simulink model "Battery_Module_To_FullPack_Grouped"  (R2024b)
settings: Solver=ode23t  StartTime=0.0  StopTime=900  MaxStep=0.05  RelTol=1e-3  AbsTol=1e-3
InitFcn:
  | % Parameters
  | vec_coolant_T=module_LUTthermalData{1};
  | vec_coolant_F=module_LUTthermalData{2};
  | mat_cellQ=module_LUTthermalData{3};
  | FlwR=coolantMassFlowRate/max(vec_coolant_F);
  | FlwT=coolantTemp-ambientTemp;
undefined symbols (not defined in the file): airGapBetweenModuleLarge, airGapBetweenModuleSmall, battery_cellH, battery_cellT, battery_cellW, battery_Np, battery_Ns, endPlateThickness
libraries: fl_lib x56, nesl_utility x14, batteryModule_lib x6
(part 1 of 2)
Description:
  | Battery Pack Thermal Management
  | 
  | Copyright 2020-2024 The MathWorks, Inc.
settings Model: Creator=vikrants  LastModifiedBy=smiller
settings SolverCC: AutoScaleAbsTol=off  AlgebraicLoopSolver=TrustRegion
settings DataIOCC: ReturnWorkspaceOutputs=off  SignalLoggingName=logsout_Battery_Module_To_FullPack_Grouped
settings DebuggingCC: UnconnectedInputMsg=warning  UnconnectedOutputMsg=warning  UnconnectedLineMsg=warning  SymbolicDimsDataTypeCodeGenerationDiagnostic=none
settings ModelReferenceCC: EnableRefExpFcnMdlSchedulingChecks=on
settings SFSimCC: CustomCodeUndefinedFunction=UseInterfaceOnly
settings RTWCC: GPUComputeCapability=3.5  DLArmComputeVersion=19.05
settings SimscapeCC: SimscapeLogType=all  SimscapeLogSimulationStatistics=on  SimscapeLogName=simlog_Battery_Module_To_FullPack_Grouped  SimscapeLogDataHistory=250000

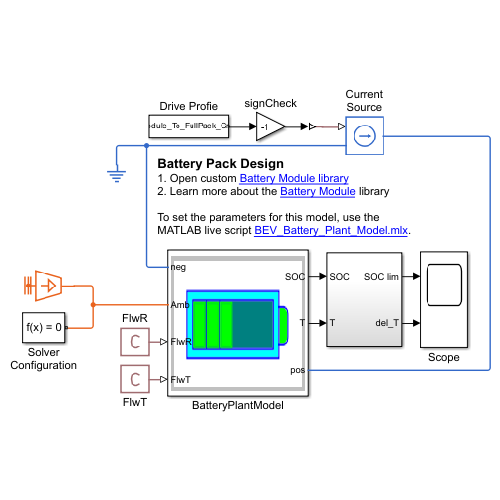
[thumbnail: Simulink's stored preview of the top-level diagram]
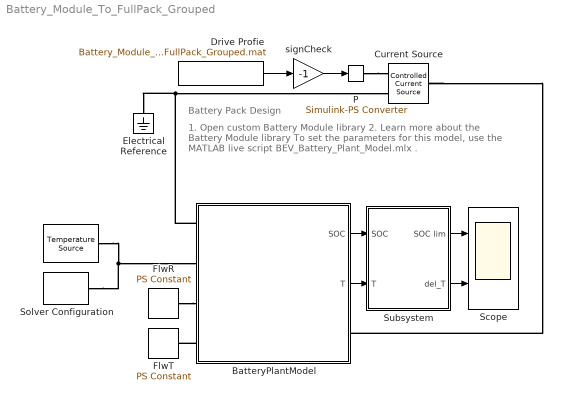
== system Battery_Module_To_FullPack_Grouped ==
  note: 1. Open custom Battery Module library
      | 2. Learn more about the Battery Module library
      |
      | To set the parameters for this model, use the
      | MATLAB live script BEV_Battery_Plant_Model.mlx .
  note: Battery Pack Design
  " " : fl_lib/Thermal/Thermal Sources/Temperature Source  temperature=ambientTemp K
  BatteryPlantModel : Subsystem
      mask Display: image('EV_Thermal_Management_BatteryIcon.png'); % Use "Edit Image" on toolstrip to change.
  Current Source : fl_lib/Electrical/Electrical Sources/Controlled Current Source
  Drive Profie : FromFile  FileName=Battery_Module_To_FullPack_Grouped.mat  SampleTime=0
  Electrical Reference : fl_lib/Electrical/Electrical Elements/Electrical Reference
  FlwR : fl_lib/Physical Signals/Sources/PS Constant  constant=FlwR
  FlwT : fl_lib/Physical Signals/Sources/PS Constant  constant=FlwT K
  P : nesl_utility/Simulink-PS Converter  PhysicalDomain=network_engine_domain  SubClassName=ps_input  LeftPortType=input  RightPortType=output  PseudoPeriodic=off  Frequencies=[]  NoiseDistribution=none  NoiseParameters=[]  Unit=A  AffineConversion=off  FilteringAndDerivatives=provide  SimscapeFilterOrder=1  InputFilterTimeConstant=0.001  UdotUserProvided=0
  Scope : Scope  NumInputPorts=2
  Solver Configuration : nesl_utility/Solver Configuration  PhysicalDomain=network_engine_domain  SubClassName=solver  LeftPortType=input  RightPortType=generic  Tones=[]  Harmonics=[]  SimulateNoise=off  Profile=off  UseLocalSampling=off  EnableSwitchedLinearOptims=on  FrequencyDomain=off  UseCCode=off  RelTol=0.001  AbsTol=1e-06  MinStep=1e-09  ToWorkspace=off  RevertToSquareIcSolve=off  NumHomotopyIterations=100  PhasorMode=off  PhasorModeNumHarmonics=1  ConsistencySolver=NEWTON_FTOL  IndexReductionMethod=DerivativeReplacement  DoDC=off  ResidualTolerance=1e-09  ConsistencyTolSource=GLOBAL  ConsistencyAbsTol=0.001  ConsistencyRelTol=0.001  ConsistencyTolFactor=0.001  UseLocalSolver=off  LocalSolverChoice=NE_BACKWARD_EULER_ADVANCER  ResolveIndetEquations=on  FunctionEvalNumThread=1  LocalSolverSampleTime=0.001  DoFixedCost=off  MaxNonlinIter=3  MaxModeIter=2  ComputeImpulses=off  ImpulseIterations=2  LinearAlgebra=auto  LinearAlgebraNumThread=0  EquationFormulation=NE_TIME_EF  DelaysMemoryBudget=1024  AutomaticFiltering=on  FilteringTimeConstant=0.001  PartitionStorageMethod=AS_NEEDED  PartitionMemoryBudget=1024  PartitionMethod=ROBUST  MultibodyUseLocalSolver=off  MultibodyLocalSolverChoice=ODE1  MultibodyLocalSolverSampleTime=0.001
  Subsystem : Subsystem
  signCheck : Gain  Gain=-1
  wires:
  Drive Profie/1 -> signCheck/1
  Subsystem/1(SOC lim) -> Scope/1
  Subsystem/2(del_T) -> Scope/2
  BatteryPlantModel/1(SOC) -> Subsystem/1(SOC)
  BatteryPlantModel/2(T) -> Subsystem/2(T)
  signCheck/1 -> P/1
  connections:
  P/RConn1 -- Current Source/RConn1
  BatteryPlantModel/LConn1 -- Electrical Reference/LConn1 -- Current Source/RConn2
  Current Source/LConn1 -- BatteryPlantModel/RConn1
  FlwR/RConn1 -- BatteryPlantModel/LConn3
  BatteryPlantModel/LConn4 -- FlwT/RConn1
  " "/LConn1 -- BatteryPlantModel/LConn2 -- Solver Configuration/RConn1

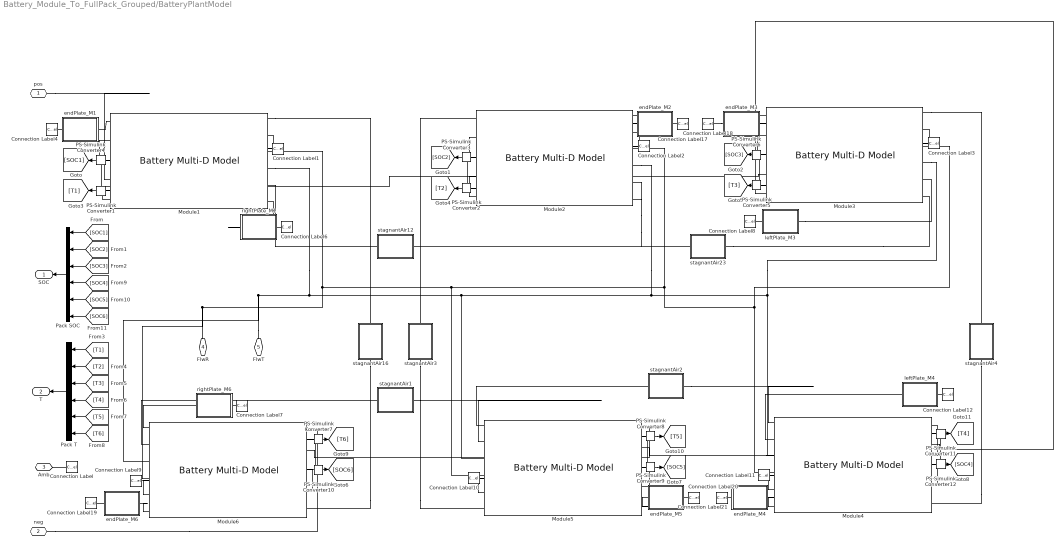
== system Battery_Module_To_FullPack_Grouped/BatteryPlantModel ==
  Connection Label{,1..4,6..12,17..21} (17 alike) : ConnectionLabel  Label=amb
  Module1 : batteryModule_lib/Battery Multi-D Model  modelComplexity=batteryModule.batteryAbstractionLevel.grouped  LUTpointsTemp=battery_vecT K  cellAH=battery_Ahr A*hr  LUTpointsSOC=battery_vecSOC  V0_mat=battery_V0 V  prm_dir=ee.enum.battery.prm_dir.noCurrentDirectionality  R0_mat=battery_R0 Ohm  R0_dis_mat=[.03, .015, .002; .04, .017, .008; .039, .012, .006; .027, .013, .021] Ohm  R0_ch_mat=[.03, .015, .002; .04, .017, .008; .039, .012, .006; .027, .013, .021] Ohm  prm_leak=ee.enum.battery.prm_leak.disabled  Rleak_vec=[8000, 7000, 6000] Ohm  extrapolation_option=simscape.enum.extrapolation.linear  prm_dyn=ee.enum.battery.prm_dyn.rc2  R1_mat=battery_R1 Ohm  tau1_mat=battery_Tau1 s  R2_mat=battery_R2 Ohm  tau2_mat=battery_Tau2 s  R3_mat=[.014, .382, .407; .028, .006, .007; .014, .007, .006; .333, .956, .912] Ohm  tau3_mat=[1, 44, 5644; 11, 24, 506; 2, 14, 330; 3310, 13419, 30216] s  R4_mat=[.014, .382, .407; .028, .006, .007; .014, .007, .006; .333, .956, .912] Ohm  tau4_mat=[1, 44, 5644; 11, 24, 506; 2, 14, 330; 3310, 13419, 30216] s  R5_mat=[.014, .382, .407; .028, .006, .007; .014, .007, .006; .333, .956, .912] Ohm  tau5_mat=[1, 44, 5644; 11, 24, 506; 2, 14, 330; 3310, 13419, 30216] s  prm_fade=ee.enum.battery.prm_fade.equations  N0=100  dV0=0  dR0=0  dAH=0  dRleak=0  dR1=0  dR2=0  dR3=0  dR4=0  dR5=0  N0vec=[100, 200, 300]  Tfadevec=[298.15, 323.15] K  dV0vec=[0, 0, 0]  dR0vec=[0, 0, 0]  dAHvec=[0, 0, 0]  dRleakvec=[0, 0, 0]  dR1vec=[0, 0, 0]  dR2vec=[0, 0, 0]  dR3vec=[0, 0, 0]  dR4vec=[0, 0, 0]  dR5vec=[0, 0, 0]  dV0mat=[0, 0; 0, 0; 0, 0]  dR0mat=[0, 0; 0, 0; 0, 0]  dAHmat=[0, 0; 0, 0; 0, 0]  dRleakmat=[0, 0; 0, 0; 0, 0]  dR1mat=[0, 0; 0, 0; 0, 0]  dR2mat=[0, 0; 0, 0; 0, 0]  dR3mat=[0, 0; 0, 0; 0, 0]  dR4mat=[0, 0; 0, 0; 0, 0]  dR5mat=[0, 0; 0, 0; 0, 0]  cellThermalMass=battery_thermalMass J/K  cellThermalCond=battery_thermalK_thru W/(m*K)  cellThermalCond_inPlane=battery_thermalK_in W/(m*K)  Ns=battery_Ns  Np=battery_Np  cellTypeSelection=batteryModule.batteryTypeSelection.pouch  cellHeight=battery_cellH m  cellWidth=battery_cellW m  cellThickness=battery_cellT m  cellDiameter=0.018 m  cellCylinLine=3  moduleExternalR=battery_extR Ohm  moduleCellBalancing=batteryModule.batteryCellBalancing.none  passiveShuntR=50 Ohm  passiveSWclosedR=0.01 Ohm  passiveSWopenCond=1e-8 1/Ohm  passiveSWthreshold=0.5  moduleCellVoltages=batteryModule.batteryCellVoltages.no  thermalManagement=batteryModule.batteryCoolingSystem.thermalPort  cellHeatTrCoeff=1 W/(m^2 * K)  thermal_moduleBottom=batteryModule.batteryThermalPortSelection.thermalLUT  htc_bottom=1 W/(m^2 * K)  moduleCooling_b=mat_cellQ W/K  LUTpointsFlowrate_b=vec_coolant_F kg/s  LUTpointsTemp_b=vec_coolant_T K  thermal_moduleTop=batteryModule.batteryThermalPortSelection.convectionBC  htc_top=battery_sidesHTC W/(m^2 * K)  moduleCooling_t=zeros(3, 6, 10) W/K  LUTpointsFlowrate_t=[.01, .02, .03, .04, .05, .06] kg/s  LUTpointsTemp_t=[273.15, 298.15, 323.15] K  thermal_moduleRight=batteryModule.batteryThermalPortSelection.thermalPortLumped  htc_right=battery_sidesHTC W/(m^2 * K)  moduleCooling_r=zeros(3, 6, 10) W/K  LUTpointsFlowrate_r=[.01, .02, .03, .04, .05, .06] kg/s  LUTpointsTemp_r=[273.15, 298.15, 323.15] K  thermal_moduleLeft=batteryModule.batteryThermalPortSelection.thermalPortLumped  htc_left=battery_sidesHTC W/(m^2 * K)  moduleCooling_l=zeros(3, 6, 10) W/K  LUTpointsFlowrate_l=[.01, .02, .03, .04, .05, .06] kg/s  LUTpointsTemp_l=[273.15, 298.15, 323.15] K  thermal_modulePos=batteryModule.batteryThermalPortSelection.thermalPortLumped  htc_pos=battery_sidesHTC W/(m^2 * K)  moduleCooling_p=zeros(3, 6, 10) W/K  LUTpointsFlowrate_p=[.01, .02, .03, .04, .05, .06] kg/s  LUTpointsTemp_p=[273.15, 298.15, 323.15] K  thermal_moduleNeg=batteryModule.batteryThermalPortSelection.thermalPortLumped  htc_neg=battery_sidesHTC W/(m^2 * K)  moduleCooling_n=zeros(3, 6, 10) W/K  LUTpointsFlowrate_n=[.01, .02, .03, .04, .05, .06] kg/s  LUTpointsTemp_n=[273.15, 298.15, 323.15] K  moduleExtHeat=battery_extHeat W  cellTemp=battery_iniT K  cellSOC=battery_iniSOC  moduleCellAHpercentVar=battery_varAhr_M1  moduleCellLeakPercentVar=ones(1, 10)  moduleCellR0PercentVar=battery_varR0_M1
      settings: InternalSimscapePortConfiguration="{\"Bottom\":[{\"id\":\"Ql\",\"label\":\"Ql\",\"type\":\"foundation.thermal.thermal\"},{\"id\":\"Qr\",\"label\":\"Qr\",\"type\":\"foundation.thermal.thermal\"}],\"Left\":[{\"id\":\"Qp\",\"label\":\"Qp\",\"type\":\"foundation.thermal.thermal\"},{\"id\":\"outputCellSOC\",\"label\":\"SOC\",\"type\":\"output\"},{\"id\":\"outputCellTemp\",\"label\":\"Temp\",\"type\":\"output\"}],\"Right\":[{\"id\":\"Qn\",\"label\":\"Qn\",\"type\":\"foundation.thermal.thermal\"},{\"id\":\"H\",\"label\":\"Amb\",\"type\":\"foundation.thermal.thermal\"},{\"id\":\"frac_b\",\"label\":\"FlwR\",\"type\":\"input\"},{\"id\":\"delT_b\",\"label\":\"FlwT\",\"type\":\"input\"}],\"Top\":[{\"id\":\"p\",\"label\":\"pos\",\"type\":\"foundation.electrical.electrical\"},{\"id\":\"n\",\"label\":\"neg\",\"type\":\"foundation.electrical.electrical\"}]}"
  Module2 : batteryModule_lib/Battery Multi-D Model  modelComplexity=batteryModule.batteryAbstractionLevel.grouped  LUTpointsTemp=battery_vecT K  cellAH=battery_Ahr A*hr  LUTpointsSOC=battery_vecSOC  V0_mat=battery_V0 V  prm_dir=ee.enum.battery.prm_dir.noCurrentDirectionality  R0_mat=battery_R0 Ohm  R0_dis_mat=[.03, .015, .002; .04, .017, .008; .039, .012, .006; .027, .013, .021] Ohm  R0_ch_mat=[.03, .015, .002; .04, .017, .008; .039, .012, .006; .027, .013, .021] Ohm  prm_leak=ee.enum.battery.prm_leak.disabled  Rleak_vec=[8000, 7000, 6000] Ohm  extrapolation_option=simscape.enum.extrapolation.linear  prm_dyn=ee.enum.battery.prm_dyn.rc2  R1_mat=battery_R1 Ohm  tau1_mat=battery_Tau1 s  R2_mat=battery_R2 Ohm  tau2_mat=battery_Tau2 s  R3_mat=[.014, .382, .407; .028, .006, .007; .014, .007, .006; .333, .956, .912] Ohm  tau3_mat=[1, 44, 5644; 11, 24, 506; 2, 14, 330; 3310, 13419, 30216] s  R4_mat=[.014, .382, .407; .028, .006, .007; .014, .007, .006; .333, .956, .912] Ohm  tau4_mat=[1, 44, 5644; 11, 24, 506; 2, 14, 330; 3310, 13419, 30216] s  R5_mat=[.014, .382, .407; .028, .006, .007; .014, .007, .006; .333, .956, .912] Ohm  tau5_mat=[1, 44, 5644; 11, 24, 506; 2, 14, 330; 3310, 13419, 30216] s  prm_fade=ee.enum.battery.prm_fade.equations  N0=100  dV0=0  dR0=0  dAH=0  dRleak=0  dR1=0  dR2=0  dR3=0  dR4=0  dR5=0  N0vec=[100, 200, 300]  Tfadevec=[298.15, 323.15] K  dV0vec=[0, 0, 0]  dR0vec=[0, 0, 0]  dAHvec=[0, 0, 0]  dRleakvec=[0, 0, 0]  dR1vec=[0, 0, 0]  dR2vec=[0, 0, 0]  dR3vec=[0, 0, 0]  dR4vec=[0, 0, 0]  dR5vec=[0, 0, 0]  dV0mat=[0, 0; 0, 0; 0, 0]  dR0mat=[0, 0; 0, 0; 0, 0]  dAHmat=[0, 0; 0, 0; 0, 0]  dRleakmat=[0, 0; 0, 0; 0, 0]  dR1mat=[0, 0; 0, 0; 0, 0]  dR2mat=[0, 0; 0, 0; 0, 0]  dR3mat=[0, 0; 0, 0; 0, 0]  dR4mat=[0, 0; 0, 0; 0, 0]  dR5mat=[0, 0; 0, 0; 0, 0]  cellThermalMass=battery_thermalMass J/K  cellThermalCond=battery_thermalK_thru W/(m*K)  cellThermalCond_inPlane=battery_thermalK_in W/(m*K)  Ns=battery_Ns  Np=battery_Np  cellTypeSelection=batteryModule.batteryTypeSelection.pouch  cellHeight=battery_cellH m  cellWidth=battery_cellW m  cellThickness=battery_cellT m  cellDiameter=0.018 m  cellCylinLine=3  moduleExternalR=battery_extR Ohm  moduleCellBalancing=batteryModule.batteryCellBalancing.none  passiveShuntR=50 Ohm  passiveSWclosedR=0.01 Ohm  passiveSWopenCond=1e-8 1/Ohm  passiveSWthreshold=0.5  moduleCellVoltages=batteryModule.batteryCellVoltages.no  thermalManagement=batteryModule.batteryCoolingSystem.thermalPort  cellHeatTrCoeff=1 W/(m^2 * K)  thermal_moduleBottom=batteryModule.batteryThermalPortSelection.thermalLUT  htc_bottom=1 W/(m^2 * K)  moduleCooling_b=mat_cellQ W/K  LUTpointsFlowrate_b=vec_coolant_F kg/s  LUTpointsTemp_b=vec_coolant_T K  thermal_moduleTop=batteryModule.batteryThermalPortSelection.convectionBC  htc_top=battery_sidesHTC W/(m^2 * K)  moduleCooling_t=zeros(3, 6, 10) W/K  LUTpointsFlowrate_t=[.01, .02, .03, .04, .05, .06] kg/s  LUTpointsTemp_t=[273.15, 298.15, 323.15] K  thermal_moduleRight=batteryModule.batteryThermalPortSelection.thermalPortLumped  htc_right=battery_sidesHTC W/(m^2 * K)  moduleCooling_r=zeros(3, 6, 10) W/K  LUTpointsFlowrate_r=[.01, .02, .03, .04, .05, .06] kg/s  LUTpointsTemp_r=[273.15, 298.15, 323.15] K  thermal_moduleLeft=batteryModule.batteryThermalPortSelection.thermalPortLumped  htc_left=battery_sidesHTC W/(m^2 * K)  moduleCooling_l=zeros(3, 6, 10) W/K  LUTpointsFlowrate_l=[.01, .02, .03, .04, .05, .06] kg/s  LUTpointsTemp_l=[273.15, 298.15, 323.15] K  thermal_modulePos=batteryModule.batteryThermalPortSelection.thermalPortLumped  htc_pos=battery_sidesHTC W/(m^2 * K)  moduleCooling_p=zeros(3, 6, 10) W/K  LUTpointsFlowrate_p=[.01, .02, .03, .04, .05, .06] kg/s  LUTpointsTemp_p=[273.15, 298.15, 323.15] K  thermal_moduleNeg=batteryModule.batteryThermalPortSelection.thermalPortLumped  htc_neg=battery_sidesHTC W/(m^2 * K)  moduleCooling_n=zeros(3, 6, 10) W/K  LUTpointsFlowrate_n=[.01, .02, .03, .04, .05, .06] kg/s  LUTpointsTemp_n=[273.15, 298.15, 323.15] K  moduleExtHeat=battery_extHeat W  cellTemp=battery_iniT K  cellSOC=battery_iniSOC  moduleCellAHpercentVar=battery_varAhr_M2  moduleCellLeakPercentVar=ones(1, 10)  moduleCellR0PercentVar=battery_varR0_M2
      settings: InternalSimscapePortConfiguration="{\"Bottom\":[{\"id\":\"Ql\",\"label\":\"Ql\",\"type\":\"foundation.thermal.thermal\"},{\"id\":\"Qr\",\"label\":\"Qr\",\"type\":\"foundation.thermal.thermal\"}],\"Left\":[{\"id\":\"Qp\",\"label\":\"Qp\",\"type\":\"foundation.thermal.thermal\"},{\"id\":\"outputCellSOC\",\"label\":\"SOC\",\"type\":\"output\"},{\"id\":\"outputCellTemp\",\"label\":\"Temp\",\"type\":\"output\"}],\"Right\":[{\"id\":\"Qn\",\"label\":\"Qn\",\"type\":\"foundation.thermal.thermal\"},{\"id\":\"H\",\"label\":\"Amb\",\"type\":\"foundation.thermal.thermal\"},{\"id\":\"frac_b\",\"label\":\"FlwR\",\"type\":\"input\"},{\"id\":\"delT_b\",\"label\":\"FlwT\",\"type\":\"input\"}],\"Top\":[{\"id\":\"p\",\"label\":\"pos\",\"type\":\"foundation.electrical.electrical\"},{\"id\":\"n\",\"label\":\"neg\",\"type\":\"foundation.electrical.electrical\"}]}"
  Module3 : batteryModule_lib/Battery Multi-D Model  modelComplexity=batteryModule.batteryAbstractionLevel.grouped  LUTpointsTemp=battery_vecT K  cellAH=battery_Ahr A*hr  LUTpointsSOC=battery_vecSOC  V0_mat=battery_V0 V  prm_dir=ee.enum.battery.prm_dir.noCurrentDirectionality  R0_mat=battery_R0 Ohm  R0_dis_mat=[.03, .015, .002; .04, .017, .008; .039, .012, .006; .027, .013, .021] Ohm  R0_ch_mat=[.03, .015, .002; .04, .017, .008; .039, .012, .006; .027, .013, .021] Ohm  prm_leak=ee.enum.battery.prm_leak.disabled  Rleak_vec=[8000, 7000, 6000] Ohm  extrapolation_option=simscape.enum.extrapolation.linear  prm_dyn=ee.enum.battery.prm_dyn.rc2  R1_mat=battery_R1 Ohm  tau1_mat=battery_Tau1 s  R2_mat=battery_R2 Ohm  tau2_mat=battery_Tau2 s  R3_mat=[.014, .382, .407; .028, .006, .007; .014, .007, .006; .333, .956, .912] Ohm  tau3_mat=[1, 44, 5644; 11, 24, 506; 2, 14, 330; 3310, 13419, 30216] s  R4_mat=[.014, .382, .407; .028, .006, .007; .014, .007, .006; .333, .956, .912] Ohm  tau4_mat=[1, 44, 5644; 11, 24, 506; 2, 14, 330; 3310, 13419, 30216] s  R5_mat=[.014, .382, .407; .028, .006, .007; .014, .007, .006; .333, .956, .912] Ohm  tau5_mat=[1, 44, 5644; 11, 24, 506; 2, 14, 330; 3310, 13419, 30216] s  prm_fade=ee.enum.battery.prm_fade.equations  N0=100  dV0=0  dR0=0  dAH=0  dRleak=0  dR1=0  dR2=0  dR3=0  dR4=0  dR5=0  N0vec=[100, 200, 300]  Tfadevec=[298.15, 323.15] K  dV0vec=[0, 0, 0]  dR0vec=[0, 0, 0]  dAHvec=[0, 0, 0]  dRleakvec=[0, 0, 0]  dR1vec=[0, 0, 0]  dR2vec=[0, 0, 0]  dR3vec=[0, 0, 0]  dR4vec=[0, 0, 0]  dR5vec=[0, 0, 0]  dV0mat=[0, 0; 0, 0; 0, 0]  dR0mat=[0, 0; 0, 0; 0, 0]  dAHmat=[0, 0; 0, 0; 0, 0]  dRleakmat=[0, 0; 0, 0; 0, 0]  dR1mat=[0, 0; 0, 0; 0, 0]  dR2mat=[0, 0; 0, 0; 0, 0]  dR3mat=[0, 0; 0, 0; 0, 0]  dR4mat=[0, 0; 0, 0; 0, 0]  dR5mat=[0, 0; 0, 0; 0, 0]  cellThermalMass=battery_thermalMass J/K  cellThermalCond=battery_thermalK_thru W/(m*K)  cellThermalCond_inPlane=battery_thermalK_in W/(m*K)  Ns=battery_Ns  Np=battery_Np  cellTypeSelection=batteryModule.batteryTypeSelection.pouch  cellHeight=battery_cellH m  cellWidth=battery_cellW m  cellThickness=battery_cellT m  cellDiameter=0.018 m  cellCylinLine=3  moduleExternalR=battery_extR Ohm  moduleCellBalancing=batteryModule.batteryCellBalancing.none  passiveShuntR=50 Ohm  passiveSWclosedR=0.01 Ohm  passiveSWopenCond=1e-8 1/Ohm  passiveSWthreshold=0.5  moduleCellVoltages=batteryModule.batteryCellVoltages.no  thermalManagement=batteryModule.batteryCoolingSystem.thermalPort  cellHeatTrCoeff=1 W/(m^2 * K)  thermal_moduleBottom=batteryModule.batteryThermalPortSelection.thermalLUT  htc_bottom=1 W/(m^2 * K)  moduleCooling_b=mat_cellQ W/K  LUTpointsFlowrate_b=vec_coolant_F kg/s  LUTpointsTemp_b=vec_coolant_T K  thermal_moduleTop=batteryModule.batteryThermalPortSelection.convectionBC  htc_top=battery_sidesHTC W/(m^2 * K)  moduleCooling_t=zeros(3, 6, 10) W/K  LUTpointsFlowrate_t=[.01, .02, .03, .04, .05, .06] kg/s  LUTpointsTemp_t=[273.15, 298.15, 323.15] K  thermal_moduleRight=batteryModule.batteryThermalPortSelection.thermalPortLumped  htc_right=battery_sidesHTC W/(m^2 * K)  moduleCooling_r=zeros(3, 6, 10) W/K  LUTpointsFlowrate_r=[.01, .02, .03, .04, .05, .06] kg/s  LUTpointsTemp_r=[273.15, 298.15, 323.15] K  thermal_moduleLeft=batteryModule.batteryThermalPortSelection.thermalPortLumped  htc_left=battery_sidesHTC W/(m^2 * K)  moduleCooling_l=zeros(3, 6, 10) W/K  LUTpointsFlowrate_l=[.01, .02, .03, .04, .05, .06] kg/s  LUTpointsTemp_l=[273.15, 298.15, 323.15] K  thermal_modulePos=batteryModule.batteryThermalPortSelection.thermalPortLumped  htc_pos=battery_sidesHTC W/(m^2 * K)  moduleCooling_p=zeros(3, 6, 10) W/K  LUTpointsFlowrate_p=[.01, .02, .03, .04, .05, .06] kg/s  LUTpointsTemp_p=[273.15, 298.15, 323.15] K  thermal_moduleNeg=batteryModule.batteryThermalPortSelection.thermalPortLumped  htc_neg=battery_sidesHTC W/(m^2 * K)  moduleCooling_n=zeros(3, 6, 10) W/K  LUTpointsFlowrate_n=[.01, .02, .03, .04, .05, .06] kg/s  LUTpointsTemp_n=[273.15, 298.15, 323.15] K  moduleExtHeat=battery_extHeat W  cellTemp=battery_iniT K  cellSOC=battery_iniSOC  moduleCellAHpercentVar=battery_varAhr_M3  moduleCellLeakPercentVar=ones(1, 10)  moduleCellR0PercentVar=battery_varR0_M3
      settings: InternalSimscapePortConfiguration="{\"Bottom\":[{\"id\":\"Ql\",\"label\":\"Ql\",\"type\":\"foundation.thermal.thermal\"},{\"id\":\"Qr\",\"label\":\"Qr\",\"type\":\"foundation.thermal.thermal\"}],\"Left\":[{\"id\":\"Qp\",\"label\":\"Qp\",\"type\":\"foundation.thermal.thermal\"},{\"id\":\"outputCellSOC\",\"label\":\"SOC\",\"type\":\"output\"},{\"id\":\"outputCellTemp\",\"label\":\"Temp\",\"type\":\"output\"}],\"Right\":[{\"id\":\"Qn\",\"label\":\"Qn\",\"type\":\"foundation.thermal.thermal\"},{\"id\":\"H\",\"label\":\"Amb\",\"type\":\"foundation.thermal.thermal\"},{\"id\":\"frac_b\",\"label\":\"FlwR\",\"type\":\"input\"},{\"id\":\"delT_b\",\"label\":\"FlwT\",\"type\":\"input\"}],\"Top\":[{\"id\":\"p\",\"label\":\"pos\",\"type\":\"foundation.electrical.electrical\"},{\"id\":\"n\",\"label\":\"neg\",\"type\":\"foundation.electrical.electrical\"}]}"
  Module4 : batteryModule_lib/Battery Multi-D Model  modelComplexity=batteryModule.batteryAbstractionLevel.grouped  LUTpointsTemp=battery_vecT K  cellAH=battery_Ahr A*hr  LUTpointsSOC=battery_vecSOC  V0_mat=battery_V0 V  prm_dir=ee.enum.battery.prm_dir.noCurrentDirectionality  R0_mat=battery_R0 Ohm  R0_dis_mat=[.03, .015, .002; .04, .017, .008; .039, .012, .006; .027, .013, .021] Ohm  R0_ch_mat=[.03, .015, .002; .04, .017, .008; .039, .012, .006; .027, .013, .021] Ohm  prm_leak=ee.enum.battery.prm_leak.disabled  Rleak_vec=[8000, 7000, 6000] Ohm  extrapolation_option=simscape.enum.extrapolation.linear  prm_dyn=ee.enum.battery.prm_dyn.rc2  R1_mat=battery_R1 Ohm  tau1_mat=battery_Tau1 s  R2_mat=battery_R2 Ohm  tau2_mat=battery_Tau2 s  R3_mat=[.014, .382, .407; .028, .006, .007; .014, .007, .006; .333, .956, .912] Ohm  tau3_mat=[1, 44, 5644; 11, 24, 506; 2, 14, 330; 3310, 13419, 30216] s  R4_mat=[.014, .382, .407; .028, .006, .007; .014, .007, .006; .333, .956, .912] Ohm  tau4_mat=[1, 44, 5644; 11, 24, 506; 2, 14, 330; 3310, 13419, 30216] s  R5_mat=[.014, .382, .407; .028, .006, .007; .014, .007, .006; .333, .956, .912] Ohm  tau5_mat=[1, 44, 5644; 11, 24, 506; 2, 14, 330; 3310, 13419, 30216] s  prm_fade=ee.enum.battery.prm_fade.equations  N0=100  dV0=0  dR0=0  dAH=0  dRleak=0  dR1=0  dR2=0  dR3=0  dR4=0  dR5=0  N0vec=[100, 200, 300]  Tfadevec=[298.15, 323.15] K  dV0vec=[0, 0, 0]  dR0vec=[0, 0, 0]  dAHvec=[0, 0, 0]  dRleakvec=[0, 0, 0]  dR1vec=[0, 0, 0]  dR2vec=[0, 0, 0]  dR3vec=[0, 0, 0]  dR4vec=[0, 0, 0]  dR5vec=[0, 0, 0]  dV0mat=[0, 0; 0, 0; 0, 0]  dR0mat=[0, 0; 0, 0; 0, 0]  dAHmat=[0, 0; 0, 0; 0, 0]  dRleakmat=[0, 0; 0, 0; 0, 0]  dR1mat=[0, 0; 0, 0; 0, 0]  dR2mat=[0, 0; 0, 0; 0, 0]  dR3mat=[0, 0; 0, 0; 0, 0]  dR4mat=[0, 0; 0, 0; 0, 0]  dR5mat=[0, 0; 0, 0; 0, 0]  cellThermalMass=battery_thermalMass J/K  cellThermalCond=battery_thermalK_thru W/(m*K)  cellThermalCond_inPlane=battery_thermalK_in W/(m*K)  Ns=battery_Ns  Np=battery_Np  cellTypeSelection=batteryModule.batteryTypeSelection.pouch  cellHeight=battery_cellH m  cellWidth=battery_cellW m  cellThickness=battery_cellT m  cellDiameter=0.018 m  cellCylinLine=3  moduleExternalR=battery_extR Ohm  moduleCellBalancing=batteryModule.batteryCellBalancing.none  passiveShuntR=50 Ohm  passiveSWclosedR=0.01 Ohm  passiveSWopenCond=1e-8 1/Ohm  passiveSWthreshold=0.5  moduleCellVoltages=batteryModule.batteryCellVoltages.no  thermalManagement=batteryModule.batteryCoolingSystem.thermalPort  cellHeatTrCoeff=1 W/(m^2 * K)  thermal_moduleBottom=batteryModule.batteryThermalPortSelection.thermalLUT  htc_bottom=1 W/(m^2 * K)  moduleCooling_b=mat_cellQ W/K  LUTpointsFlowrate_b=vec_coolant_F kg/s  LUTpointsTemp_b=vec_coolant_T K  thermal_moduleTop=batteryModule.batteryThermalPortSelection.convectionBC  htc_top=battery_sidesHTC W/(m^2 * K)  moduleCooling_t=zeros(3, 6, 10) W/K  LUTpointsFlowrate_t=[.01, .02, .03, .04, .05, .06] kg/s  LUTpointsTemp_t=[273.15, 298.15, 323.15] K  thermal_moduleRight=batteryModule.batteryThermalPortSelection.thermalPortLumped  htc_right=battery_sidesHTC W/(m^2 * K)  moduleCooling_r=zeros(3, 6, 10) W/K  LUTpointsFlowrate_r=[.01, .02, .03, .04, .05, .06] kg/s  LUTpointsTemp_r=[273.15, 298.15, 323.15] K  thermal_moduleLeft=batteryModule.batteryThermalPortSelection.thermalPortLumped  htc_left=battery_sidesHTC W/(m^2 * K)  moduleCooling_l=zeros(3, 6, 10) W/K  LUTpointsFlowrate_l=[.01, .02, .03, .04, .05, .06] kg/s  LUTpointsTemp_l=[273.15, 298.15, 323.15] K  thermal_modulePos=batteryModule.batteryThermalPortSelection.thermalPortLumped  htc_pos=battery_sidesHTC W/(m^2 * K)  moduleCooling_p=zeros(3, 6, 10) W/K  LUTpointsFlowrate_p=[.01, .02, .03, .04, .05, .06] kg/s  LUTpointsTemp_p=[273.15, 298.15, 323.15] K  thermal_moduleNeg=batteryModule.batteryThermalPortSelection.thermalPortLumped  htc_neg=battery_sidesHTC W/(m^2 * K)  moduleCooling_n=zeros(3, 6, 10) W/K  LUTpointsFlowrate_n=[.01, .02, .03, .04, .05, .06] kg/s  LUTpointsTemp_n=[273.15, 298.15, 323.15] K  moduleExtHeat=battery_extHeat W  cellTemp=battery_iniT K  cellSOC=battery_iniSOC  moduleCellAHpercentVar=battery_varAhr_M4  moduleCellLeakPercentVar=ones(1, 10)  moduleCellR0PercentVar=battery_varR0_M4
      settings: InternalSimscapePortConfiguration="{\"Bottom\":[{\"id\":\"Ql\",\"label\":\"Ql\",\"type\":\"foundation.thermal.thermal\"},{\"id\":\"Qr\",\"label\":\"Qr\",\"type\":\"foundation.thermal.thermal\"}],\"Left\":[{\"id\":\"Qp\",\"label\":\"Qp\",\"type\":\"foundation.thermal.thermal\"},{\"id\":\"outputCellSOC\",\"label\":\"SOC\",\"type\":\"output\"},{\"id\":\"outputCellTemp\",\"label\":\"Temp\",\"type\":\"output\"}],\"Right\":[{\"id\":\"Qn\",\"label\":\"Qn\",\"type\":\"foundation.thermal.thermal\"},{\"id\":\"H\",\"label\":\"Amb\",\"type\":\"foundation.thermal.thermal\"},{\"id\":\"frac_b\",\"label\":\"FlwR\",\"type\":\"input\"},{\"id\":\"delT_b\",\"label\":\"FlwT\",\"type\":\"input\"}],\"Top\":[{\"id\":\"p\",\"label\":\"pos\",\"type\":\"foundation.electrical.electrical\"},{\"id\":\"n\",\"label\":\"neg\",\"type\":\"foundation.electrical.electrical\"}]}"
  Module5 : batteryModule_lib/Battery Multi-D Model  modelComplexity=batteryModule.batteryAbstractionLevel.grouped  LUTpointsTemp=battery_vecT K  cellAH=battery_Ahr A*hr  LUTpointsSOC=battery_vecSOC  V0_mat=battery_V0 V  prm_dir=ee.enum.battery.prm_dir.noCurrentDirectionality  R0_mat=battery_R0 Ohm  R0_dis_mat=[.03, .015, .002; .04, .017, .008; .039, .012, .006; .027, .013, .021] Ohm  R0_ch_mat=[.03, .015, .002; .04, .017, .008; .039, .012, .006; .027, .013, .021] Ohm  prm_leak=ee.enum.battery.prm_leak.disabled  Rleak_vec=[8000, 7000, 6000] Ohm  extrapolation_option=simscape.enum.extrapolation.linear  prm_dyn=ee.enum.battery.prm_dyn.rc2  R1_mat=battery_R1 Ohm  tau1_mat=battery_Tau1 s  R2_mat=battery_R2 Ohm  tau2_mat=battery_Tau2 s  R3_mat=[.014, .382, .407; .028, .006, .007; .014, .007, .006; .333, .956, .912] Ohm  tau3_mat=[1, 44, 5644; 11, 24, 506; 2, 14, 330; 3310, 13419, 30216] s  R4_mat=[.014, .382, .407; .028, .006, .007; .014, .007, .006; .333, .956, .912] Ohm  tau4_mat=[1, 44, 5644; 11, 24, 506; 2, 14, 330; 3310, 13419, 30216] s  R5_mat=[.014, .382, .407; .028, .006, .007; .014, .007, .006; .333, .956, .912] Ohm  tau5_mat=[1, 44, 5644; 11, 24, 506; 2, 14, 330; 3310, 13419, 30216] s  prm_fade=ee.enum.battery.prm_fade.equations  N0=100  dV0=0  dR0=0  dAH=0  dRleak=0  dR1=0  dR2=0  dR3=0  dR4=0  dR5=0  N0vec=[100, 200, 300]  Tfadevec=[298.15, 323.15] K  dV0vec=[0, 0, 0]  dR0vec=[0, 0, 0]  dAHvec=[0, 0, 0]  dRleakvec=[0, 0, 0]  dR1vec=[0, 0, 0]  dR2vec=[0, 0, 0]  dR3vec=[0, 0, 0]  dR4vec=[0, 0, 0]  dR5vec=[0, 0, 0]  dV0mat=[0, 0; 0, 0; 0, 0]  dR0mat=[0, 0; 0, 0; 0, 0]  dAHmat=[0, 0; 0, 0; 0, 0]  dRleakmat=[0, 0; 0, 0; 0, 0]  dR1mat=[0, 0; 0, 0; 0, 0]  dR2mat=[0, 0; 0, 0; 0, 0]  dR3mat=[0, 0; 0, 0; 0, 0]  dR4mat=[0, 0; 0, 0; 0, 0]  dR5mat=[0, 0; 0, 0; 0, 0]  cellThermalMass=battery_thermalMass J/K  cellThermalCond=battery_thermalK_thru W/(m*K)  cellThermalCond_inPlane=battery_thermalK_in W/(m*K)  Ns=battery_Ns  Np=battery_Np  cellTypeSelection=batteryModule.batteryTypeSelection.pouch  cellHeight=battery_cellH m  cellWidth=battery_cellW m  cellThickness=battery_cellT m  cellDiameter=0.018 m  cellCylinLine=3  moduleExternalR=battery_extR Ohm  moduleCellBalancing=batteryModule.batteryCellBalancing.none  passiveShuntR=50 Ohm  passiveSWclosedR=0.01 Ohm  passiveSWopenCond=1e-8 1/Ohm  passiveSWthreshold=0.5  moduleCellVoltages=batteryModule.batteryCellVoltages.no  thermalManagement=batteryModule.batteryCoolingSystem.thermalPort  cellHeatTrCoeff=1 W/(m^2 * K)  thermal_moduleBottom=batteryModule.batteryThermalPortSelection.thermalLUT  htc_bottom=1 W/(m^2 * K)  moduleCooling_b=mat_cellQ W/K  LUTpointsFlowrate_b=vec_coolant_F kg/s  LUTpointsTemp_b=vec_coolant_T K  thermal_moduleTop=batteryModule.batteryThermalPortSelection.convectionBC  htc_top=battery_sidesHTC W/(m^2 * K)  moduleCooling_t=zeros(3, 6, 10) W/K  LUTpointsFlowrate_t=[.01, .02, .03, .04, .05, .06] kg/s  LUTpointsTemp_t=[273.15, 298.15, 323.15] K  thermal_moduleRight=batteryModule.batteryThermalPortSelection.thermalPortLumped  htc_right=battery_sidesHTC W/(m^2 * K)  moduleCooling_r=zeros(3, 6, 10) W/K  LUTpointsFlowrate_r=[.01, .02, .03, .04, .05, .06] kg/s  LUTpointsTemp_r=[273.15, 298.15, 323.15] K  thermal_moduleLeft=batteryModule.batteryThermalPortSelection.thermalPortLumped  htc_left=battery_sidesHTC W/(m^2 * K)  moduleCooling_l=zeros(3, 6, 10) W/K  LUTpointsFlowrate_l=[.01, .02, .03, .04, .05, .06] kg/s  LUTpointsTemp_l=[273.15, 298.15, 323.15] K  thermal_modulePos=batteryModule.batteryThermalPortSelection.thermalPortLumped  htc_pos=battery_sidesHTC W/(m^2 * K)  moduleCooling_p=zeros(3, 6, 10) W/K  LUTpointsFlowrate_p=[.01, .02, .03, .04, .05, .06] kg/s  LUTpointsTemp_p=[273.15, 298.15, 323.15] K  thermal_moduleNeg=batteryModule.batteryThermalPortSelection.thermalPortLumped  htc_neg=battery_sidesHTC W/(m^2 * K)  moduleCooling_n=zeros(3, 6, 10) W/K  LUTpointsFlowrate_n=[.01, .02, .03, .04, .05, .06] kg/s  LUTpointsTemp_n=[273.15, 298.15, 323.15] K  moduleExtHeat=battery_extHeat W  cellTemp=battery_iniT K  cellSOC=battery_iniSOC  moduleCellAHpercentVar=battery_varAhr_M5  moduleCellLeakPercentVar=ones(1, 10)  moduleCellR0PercentVar=battery_varR0_M5
      settings: InternalSimscapePortConfiguration="{\"Bottom\":[{\"id\":\"Ql\",\"label\":\"Ql\",\"type\":\"foundation.thermal.thermal\"},{\"id\":\"Qr\",\"label\":\"Qr\",\"type\":\"foundation.thermal.thermal\"}],\"Left\":[{\"id\":\"Qp\",\"label\":\"Qp\",\"type\":\"foundation.thermal.thermal\"},{\"id\":\"outputCellSOC\",\"label\":\"SOC\",\"type\":\"output\"},{\"id\":\"outputCellTemp\",\"label\":\"Temp\",\"type\":\"output\"}],\"Right\":[{\"id\":\"Qn\",\"label\":\"Qn\",\"type\":\"foundation.thermal.thermal\"},{\"id\":\"H\",\"label\":\"Amb\",\"type\":\"foundation.thermal.thermal\"},{\"id\":\"frac_b\",\"label\":\"FlwR\",\"type\":\"input\"},{\"id\":\"delT_b\",\"label\":\"FlwT\",\"type\":\"input\"}],\"Top\":[{\"id\":\"p\",\"label\":\"pos\",\"type\":\"foundation.electrical.electrical\"},{\"id\":\"n\",\"label\":\"neg\",\"type\":\"foundation.electrical.electrical\"}]}"
  Module6 : batteryModule_lib/Battery Multi-D Model  modelComplexity=batteryModule.batteryAbstractionLevel.grouped  LUTpointsTemp=battery_vecT K  cellAH=battery_Ahr A*hr  LUTpointsSOC=battery_vecSOC  V0_mat=battery_V0 V  prm_dir=ee.enum.battery.prm_dir.noCurrentDirectionality  R0_mat=battery_R0 Ohm  R0_dis_mat=[.03, .015, .002; .04, .017, .008; .039, .012, .006; .027, .013, .021] Ohm  R0_ch_mat=[.03, .015, .002; .04, .017, .008; .039, .012, .006; .027, .013, .021] Ohm  prm_leak=ee.enum.battery.prm_leak.disabled  Rleak_vec=[8000, 7000, 6000] Ohm  extrapolation_option=simscape.enum.extrapolation.linear  prm_dyn=ee.enum.battery.prm_dyn.rc2  R1_mat=battery_R1 Ohm  tau1_mat=battery_Tau1 s  R2_mat=battery_R2 Ohm  tau2_mat=battery_Tau2 s  R3_mat=[.014, .382, .407; .028, .006, .007; .014, .007, .006; .333, .956, .912] Ohm  tau3_mat=[1, 44, 5644; 11, 24, 506; 2, 14, 330; 3310, 13419, 30216] s  R4_mat=[.014, .382, .407; .028, .006, .007; .014, .007, .006; .333, .956, .912] Ohm  tau4_mat=[1, 44, 5644; 11, 24, 506; 2, 14, 330; 3310, 13419, 30216] s  R5_mat=[.014, .382, .407; .028, .006, .007; .014, .007, .006; .333, .956, .912] Ohm  tau5_mat=[1, 44, 5644; 11, 24, 506; 2, 14, 330; 3310, 13419, 30216] s  prm_fade=ee.enum.battery.prm_fade.equations  N0=100  dV0=0  dR0=0  dAH=0  dRleak=0  dR1=0  dR2=0  dR3=0  dR4=0  dR5=0  N0vec=[100, 200, 300]  Tfadevec=[298.15, 323.15] K  dV0vec=[0, 0, 0]  dR0vec=[0, 0, 0]  dAHvec=[0, 0, 0]  dRleakvec=[0, 0, 0]  dR1vec=[0, 0, 0]  dR2vec=[0, 0, 0]  dR3vec=[0, 0, 0]  dR4vec=[0, 0, 0]  dR5vec=[0, 0, 0]  dV0mat=[0, 0; 0, 0; 0, 0]  dR0mat=[0, 0; 0, 0; 0, 0]  dAHmat=[0, 0; 0, 0; 0, 0]  dRleakmat=[0, 0; 0, 0; 0, 0]  dR1mat=[0, 0; 0, 0; 0, 0]  dR2mat=[0, 0; 0, 0; 0, 0]  dR3mat=[0, 0; 0, 0; 0, 0]  dR4mat=[0, 0; 0, 0; 0, 0]  dR5mat=[0, 0; 0, 0; 0, 0]  cellThermalMass=battery_thermalMass J/K  cellThermalCond=battery_thermalK_thru W/(m*K)  cellThermalCond_inPlane=battery_thermalK_in W/(m*K)  Ns=battery_Ns  Np=battery_Np  cellTypeSelection=batteryModule.batteryTypeSelection.pouch  cellHeight=battery_cellH m  cellWidth=battery_cellW m  cellThickness=battery_cellT m  cellDiameter=0.018 m  cellCylinLine=3  moduleExternalR=battery_extR Ohm  moduleCellBalancing=batteryModule.batteryCellBalancing.none  passiveShuntR=50 Ohm  passiveSWclosedR=0.01 Ohm  passiveSWopenCond=1e-8 1/Ohm  passiveSWthreshold=0.5  moduleCellVoltages=batteryModule.batteryCellVoltages.no  thermalManagement=batteryModule.batteryCoolingSystem.thermalPort  cellHeatTrCoeff=1 W/(m^2 * K)  thermal_moduleBottom=batteryModule.batteryThermalPortSelection.thermalLUT  htc_bottom=1 W/(m^2 * K)  moduleCooling_b=mat_cellQ W/K  LUTpointsFlowrate_b=vec_coolant_F kg/s  LUTpointsTemp_b=vec_coolant_T K  thermal_moduleTop=batteryModule.batteryThermalPortSelection.convectionBC  htc_top=battery_sidesHTC W/(m^2 * K)  moduleCooling_t=zeros(3, 6, 10) W/K  LUTpointsFlowrate_t=[.01, .02, .03, .04, .05, .06] kg/s  LUTpointsTemp_t=[273.15, 298.15, 323.15] K  thermal_moduleRight=batteryModule.batteryThermalPortSelection.thermalPortLumped  htc_right=battery_sidesHTC W/(m^2 * K)  moduleCooling_r=zeros(3, 6, 10) W/K  LUTpointsFlowrate_r=[.01, .02, .03, .04, .05, .06] kg/s  LUTpointsTemp_r=[273.15, 298.15, 323.15] K  thermal_moduleLeft=batteryModule.batteryThermalPortSelection.thermalPortLumped  htc_left=battery_sidesHTC W/(m^2 * K)  moduleCooling_l=zeros(3, 6, 10) W/K  LUTpointsFlowrate_l=[.01, .02, .03, .04, .05, .06] kg/s  LUTpointsTemp_l=[273.15, 298.15, 323.15] K  thermal_modulePos=batteryModule.batteryThermalPortSelection.thermalPortLumped  htc_pos=battery_sidesHTC W/(m^2 * K)  moduleCooling_p=zeros(3, 6, 10) W/K  LUTpointsFlowrate_p=[.01, .02, .03, .04, .05, .06] kg/s  LUTpointsTemp_p=[273.15, 298.15, 323.15] K  thermal_moduleNeg=batteryModule.batteryThermalPortSelection.thermalPortLumped  htc_neg=battery_sidesHTC W/(m^2 * K)  moduleCooling_n=zeros(3, 6, 10) W/K  LUTpointsFlowrate_n=[.01, .02, .03, .04, .05, .06] kg/s  LUTpointsTemp_n=[273.15, 298.15, 323.15] K  moduleExtHeat=battery_extHeat W  cellTemp=battery_iniT K  cellSOC=battery_iniSOC  moduleCellAHpercentVar=battery_varAhr_M6  moduleCellLeakPercentVar=ones(1, 10)  moduleCellR0PercentVar=battery_varR0_M6
      settings: InternalSimscapePortConfiguration="{\"Bottom\":[{\"id\":\"Ql\",\"label\":\"Ql\",\"type\":\"foundation.thermal.thermal\"},{\"id\":\"Qr\",\"label\":\"Qr\",\"type\":\"foundation.thermal.thermal\"}],\"Left\":[{\"id\":\"Qp\",\"label\":\"Qp\",\"type\":\"foundation.thermal.thermal\"},{\"id\":\"outputCellSOC\",\"label\":\"SOC\",\"type\":\"output\"},{\"id\":\"outputCellTemp\",\"label\":\"Temp\",\"type\":\"output\"}],\"Right\":[{\"id\":\"Qn\",\"label\":\"Qn\",\"type\":\"foundation.thermal.thermal\"},{\"id\":\"H\",\"label\":\"Amb\",\"type\":\"foundation.thermal.thermal\"},{\"id\":\"frac_b\",\"label\":\"FlwR\",\"type\":\"input\"},{\"id\":\"delT_b\",\"label\":\"FlwT\",\"type\":\"input\"}],\"Top\":[{\"id\":\"p\",\"label\":\"pos\",\"type\":\"foundation.electrical.electrical\"},{\"id\":\"n\",\"label\":\"neg\",\"type\":\"foundation.electrical.electrical\"}]}"
  PS-Simulink Converter{1..2,5,7..8,11} (6 alike) : nesl_utility/PS-Simulink Converter  PhysicalDomain=network_engine_domain  SubClassName=ps_output  LeftPortType=input  RightPortType=output  PseudoPeriodic=off  Frequencies=[]  VectorFormat=1-D array  Unit=K  AffineConversion=on
  PS-Simulink Converter{3..4,6,9..10,12} (6 alike) : nesl_utility/PS-Simulink Converter  PhysicalDomain=network_engine_domain  SubClassName=ps_output  LeftPortType=input  RightPortType=output  PseudoPeriodic=off  Frequencies=[]  VectorFormat=1-D array  Unit=1  AffineConversion=on
  Pack SOC : Concatenate  NumInputs=6
  Pack T : Concatenate  NumInputs=6
  endPlate_M1 : Subsystem
  endPlate_M2 : Subsystem
  endPlate_M3 : Subsystem
  endPlate_M4 : Subsystem
  endPlate_M5 : Subsystem
  endPlate_M6 : Subsystem
  leftPlate_M3 : Subsystem
  leftPlate_M4 : Subsystem
  rightPlate_M1 : Subsystem
  rightPlate_M6 : Subsystem
  stagnantAir1 : Subsystem
  stagnantAir12 : Subsystem
  stagnantAir16 : Subsystem
  stagnantAir2 : Subsystem
  stagnantAir23 : Subsystem
  stagnantAir3 : Subsystem
  stagnantAir4 : Subsystem
  pos : PMIOPort  Side=Right
  neg : PMIOPort  Port=2  Side=Left
  Amb : PMIOPort  Port=3  Side=Left
  FlwR : PMIOPort  Port=4  Side=Left
  FlwT : PMIOPort  Port=5  Side=Left
  SOC : Outport
  T : Outport  Port=2
  wires:
  Pack SOC/1 -> SOC/1
  Pack T/1 -> T/1
  [SOC1] -> Pack SOC/1
  [SOC2] -> Pack SOC/2
  PS-Simulink Converter3/1 -> [SOC2]
  PS-Simulink Converter4/1 -> [SOC1]
  PS-Simulink Converter6/1 -> [SOC3]
  [SOC3] -> Pack SOC/3
  PS-Simulink Converter1/1 -> [T1]
  [T1] -> Pack T/1
  PS-Simulink Converter2/1 -> [T2]
  [T2] -> Pack T/2
  PS-Simulink Converter5/1 -> [T3]
  [T3] -> Pack T/3
  PS-Simulink Converter11/1 -> [T4]
  PS-Simulink Converter12/1 -> [SOC4]
  PS-Simulink Converter8/1 -> [T5]
  PS-Simulink Converter9/1 -> [SOC5]
  PS-Simulink Converter7/1 -> [T6]
  PS-Simulink Converter10/1 -> [SOC6]
  [T4] -> Pack T/4
  [T5] -> Pack T/5
  [T6] -> Pack T/6
  [SOC4] -> Pack SOC/4
  [SOC5] -> Pack SOC/5
  [SOC6] -> Pack SOC/6
  connections:
  Connection Label/LConn1 -- Amb/RConn1
  FlwT/RConn1 -- Module3/RConn4 -- Module4/RConn4 -- Module2/RConn4 -- Module5/RConn4 -- Module1/RConn4 -- Module6/RConn4
  Module2/RConn3 -- FlwR/RConn1 -- Module6/RConn3 -- Module1/RConn3 -- Module5/RConn3 -- Module3/RConn3 -- Module4/RConn3
  Connection Label1/LConn1 -- Module1/RConn2
  PS-Simulink Converter3/LConn1 -- Module2/LConn2
  PS-Simulink Converter2/LConn1 -- Module2/LConn3
  Connection Label2/LConn1 -- Module2/RConn2
  PS-Simulink Converter5/LConn1 -- Module3/LConn3
  PS-Simulink Converter6/LConn1 -- Module3/LConn2
  Module3/LConn4 -- Module2/LConn5
  Connection Label3/LConn1 -- Module3/RConn2
  Module1/LConn5 -- Module2/LConn4
  pos/RConn1 -- Module1/LConn4
  PS-Simulink Converter1/LConn1 -- Module1/LConn3
  PS-Simulink Converter4/LConn1 -- Module1/LConn2
  Connection Label4/LConn1 -- endPlate_M1/LConn1
  Connection Label11/LConn1 -- Module4/RConn2
  PS-Simulink Converter8/LConn1 -- Module5/LConn3
  PS-Simulink Converter10/LConn1 -- Module6/LConn2
  Connection Label9/LConn1 -- Module6/RConn2
  PS-Simulink Converter9/LConn1 -- Module5/LConn2
  PS-Simulink Converter12/LConn1 -- Module4/LConn2
  Connection Label10/LConn1 -- Module5/RConn2
  PS-Simulink Converter11/LConn1 -- Module4/LConn3
  PS-Simulink Converter7/LConn1 -- Module6/LConn3
  Module6/LConn4 -- Module5/LConn5
  neg/RConn1 -- Module6/LConn5
  Module5/LConn4 -- Module4/LConn5
  Module4/LConn4 -- Module3/LConn5
  Module1/RConn1 -- stagnantAir16/LConn1
  stagnantAir16/RConn1 -- Module6/LConn1
  endPlate_M1/RConn1 -- Module1/LConn1
  Connection Label17/LConn1 -- endPlate_M2/LConn1
  endPlate_M2/RConn1 -- Module2/RConn1
  Connection Label18/LConn1 -- endPlate_M3/LConn1
  endPlate_M3/RConn1 -- Module3/LConn1
  Connection Label19/LConn1 -- endPlate_M6/LConn1
  endPlate_M6/RConn1 -- Module6/RConn1
  Connection Label20/LConn1 -- endPlate_M5/LConn1
  Module5/LConn1 -- endPlate_M5/RConn1
  Connection Label21/LConn1 -- endPlate_M4/LConn1
  endPlate_M4/RConn1 -- Module4/RConn1
  stagnantAir3/LConn1 -- Module2/LConn1
  stagnantAir3/RConn1 -- Module5/RConn1
  Module3/RConn1 -- stagnantAir4/LConn1
  stagnantAir4/RConn1 -- Module4/LConn1
  Module1/RConn5 -- stagnantAir12/LConn1
  Module2/RConn5 -- stagnantAir12/RConn1
  Module2/RConn6 -- stagnantAir23/LConn1
  stagnantAir23/RConn1 -- Module3/RConn6
  rightPlate_M1/RConn1 -- Module1/RConn6
  leftPlate_M3/RConn1 -- Module3/RConn5
  Connection Label8/LConn1 -- leftPlate_M3/LConn1
  Connection Label6/LConn1 -- rightPlate_M1/LConn1
  Module6/RConn5 -- stagnantAir1/LConn1
  stagnantAir1/RConn1 -- Module5/RConn5
  Module5/RConn6 -- stagnantAir2/LConn1
  stagnantAir2/RConn1 -- Module4/RConn6
  rightPlate_M6/RConn1 -- Module6/RConn6
  rightPlate_M6/LConn1 -- Connection Label7/LConn1
  leftPlate_M4/LConn1 -- Connection Label12/LConn1
  leftPlate_M4/RConn1 -- Module4/RConn5

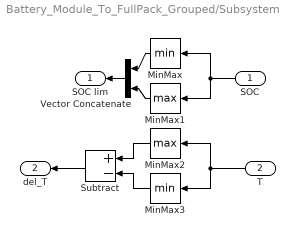
== system Battery_Module_To_FullPack_Grouped/Subsystem ==
  SOC : Inport
  T : Inport  Port=2
  MinMax : MinMax
  MinMax1 : MinMax  Function=max
  MinMax2 : MinMax  Function=max
  MinMax3 : MinMax
  Subtract : Sum  Inputs=+-
  Vector Concatenate : Concatenate
  SOC lim : Outport
  del_T : Outport  Port=2
  wires:
  MinMax/1 -> Vector Concatenate/1
  SOC/1 -> MinMax/1, MinMax1/1
  Vector Concatenate/1 -> SOC lim/1
  MinMax1/1 -> Vector Concatenate/2
  T/1 -> MinMax2/1, MinMax3/1
  MinMax2/1 -> Subtract/1
  MinMax3/1 -> Subtract/2
  Subtract/1 -> del_T/1

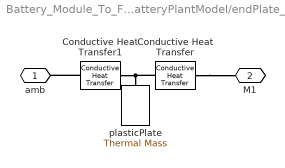
== system Battery_Module_To_FullPack_Grouped/BatteryPlantModel/endPlate_M1 ==
  Conductive Heat Transfer : fl_lib/Thermal/Thermal Elements/Conductive Heat Transfer  thermal_type=foundation.enum.ConstantVariableTabulated.Constant  wall_geometry=foundation.enum.ConductionWallGeometry.Planar  area=battery_cellH*battery_cellW m^2  thickness=endPlateThickness m  d_in=0.05 m  d_out=0.1 m  L=1 m  th_cond_min=10 W/(K*m)  th_cond=0.024 W/(m*K)  th_cond_TLU=[413, 401, 392, 383, 371, 357, 342] W/(K*m)  temp_TLU=[200, 273, 400, 600, 800, 1000, 1200] K  T_specify=off  T_priority=None  T=0 K  T_nominal_specify=off  T_nominal_value=1  T_nominal_unit=K  Q_specify=off  Q_priority=None  Q=0 W  Q_nominal_specify=off  Q_nominal_value=1  Q_nominal_unit=W
  Conductive Heat Transfer1 : fl_lib/Thermal/Thermal Elements/Conductive Heat Transfer  thermal_type=foundation.enum.ConstantVariableTabulated.Constant  wall_geometry=foundation.enum.ConductionWallGeometry.Planar  area=battery_cellH*battery_cellW m^2  thickness=endPlateThickness m  d_in=0.05 m  d_out=0.1 m  L=1 m  th_cond_min=10 W/(K*m)  th_cond=0.024 W/(m*K)  th_cond_TLU=[413, 401, 392, 383, 371, 357, 342] W/(K*m)  temp_TLU=[200, 273, 400, 600, 800, 1000, 1200] K  T_specify=off  T_priority=None  T=0 K  T_nominal_specify=off  T_nominal_value=1  T_nominal_unit=K  Q_specify=off  Q_priority=None  Q=0 W  Q_nominal_specify=off  Q_nominal_value=1  Q_nominal_unit=W
  plasticPlate : fl_lib/Thermal/Thermal Elements/Thermal Mass  mass_type=foundation.enum.constant_variable.constant  mass=battery_cellH*battery_cellW*endPlateThickness*44 kg  sp_heat=400 J/kg/K  mass_min=1e-6 kg  num_ports=foundation.enum.numPorts2.one  m_specify=off  m_priority=High  m=1 kg  m_nominal_specify=off  m_nominal_value=1  m_nominal_unit=kg  T_specify=off  T_priority=High  T=300 K  T_nominal_specify=off  T_nominal_value=1  T_nominal_unit=K  Q_specify=off  Q_priority=None  Q=0 W  Q_nominal_specify=off  Q_nominal_value=1  Q_nominal_unit=W
  amb : PMIOPort  Side=Left
  M1 : PMIOPort  Port=2  Side=Right
  connections:
  Conductive Heat Transfer1/LConn1 -- plasticPlate/LConn1 -- Conductive Heat Transfer/RConn1
  Conductive Heat Transfer/LConn1 -- M1/RConn1
  Conductive Heat Transfer1/RConn1 -- amb/RConn1

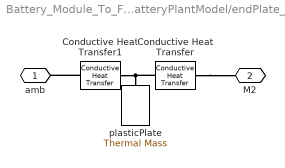
== system Battery_Module_To_FullPack_Grouped/BatteryPlantModel/endPlate_M2 ==
  Conductive Heat Transfer : fl_lib/Thermal/Thermal Elements/Conductive Heat Transfer  thermal_type=foundation.enum.ConstantVariableTabulated.Constant  wall_geometry=foundation.enum.ConductionWallGeometry.Planar  area=battery_cellH*battery_cellW m^2  thickness=endPlateThickness m  d_in=0.05 m  d_out=0.1 m  L=1 m  th_cond_min=10 W/(K*m)  th_cond=0.024 W/(m*K)  th_cond_TLU=[413, 401, 392, 383, 371, 357, 342] W/(K*m)  temp_TLU=[200, 273, 400, 600, 800, 1000, 1200] K  T_specify=off  T_priority=None  T=0 K  T_nominal_specify=off  T_nominal_value=1  T_nominal_unit=K  Q_specify=off  Q_priority=None  Q=0 W  Q_nominal_specify=off  Q_nominal_value=1  Q_nominal_unit=W
  Conductive Heat Transfer1 : fl_lib/Thermal/Thermal Elements/Conductive Heat Transfer  thermal_type=foundation.enum.ConstantVariableTabulated.Constant  wall_geometry=foundation.enum.ConductionWallGeometry.Planar  area=battery_cellH*battery_cellW m^2  thickness=endPlateThickness m  d_in=0.05 m  d_out=0.1 m  L=1 m  th_cond_min=10 W/(K*m)  th_cond=0.024 W/(m*K)  th_cond_TLU=[413, 401, 392, 383, 371, 357, 342] W/(K*m)  temp_TLU=[200, 273, 400, 600, 800, 1000, 1200] K  T_specify=off  T_priority=None  T=0 K  T_nominal_specify=off  T_nominal_value=1  T_nominal_unit=K  Q_specify=off  Q_priority=None  Q=0 W  Q_nominal_specify=off  Q_nominal_value=1  Q_nominal_unit=W
  plasticPlate : fl_lib/Thermal/Thermal Elements/Thermal Mass  mass_type=foundation.enum.constant_variable.constant  mass=battery_cellH*battery_cellW*endPlateThickness*44 kg  sp_heat=400 J/kg/K  mass_min=1e-6 kg  num_ports=foundation.enum.numPorts2.one  m_specify=off  m_priority=High  m=1 kg  m_nominal_specify=off  m_nominal_value=1  m_nominal_unit=kg  T_specify=off  T_priority=High  T=300 K  T_nominal_specify=off  T_nominal_value=1  T_nominal_unit=K  Q_specify=off  Q_priority=None  Q=0 W  Q_nominal_specify=off  Q_nominal_value=1  Q_nominal_unit=W
  amb : PMIOPort  Side=Left
  M2 : PMIOPort  Port=2  Side=Right
  connections:
  Conductive Heat Transfer1/LConn1 -- plasticPlate/LConn1 -- Conductive Heat Transfer/RConn1
  Conductive Heat Transfer/LConn1 -- M2/RConn1
  Conductive Heat Transfer1/RConn1 -- amb/RConn1

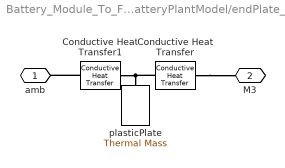
== system Battery_Module_To_FullPack_Grouped/BatteryPlantModel/endPlate_M3 ==
  Conductive Heat Transfer : fl_lib/Thermal/Thermal Elements/Conductive Heat Transfer  thermal_type=foundation.enum.ConstantVariableTabulated.Constant  wall_geometry=foundation.enum.ConductionWallGeometry.Planar  area=battery_cellH*battery_cellW m^2  thickness=endPlateThickness m  d_in=0.05 m  d_out=0.1 m  L=1 m  th_cond_min=10 W/(K*m)  th_cond=0.024 W/(m*K)  th_cond_TLU=[413, 401, 392, 383, 371, 357, 342] W/(K*m)  temp_TLU=[200, 273, 400, 600, 800, 1000, 1200] K  T_specify=off  T_priority=None  T=0 K  T_nominal_specify=off  T_nominal_value=1  T_nominal_unit=K  Q_specify=off  Q_priority=None  Q=0 W  Q_nominal_specify=off  Q_nominal_value=1  Q_nominal_unit=W
  Conductive Heat Transfer1 : fl_lib/Thermal/Thermal Elements/Conductive Heat Transfer  thermal_type=foundation.enum.ConstantVariableTabulated.Constant  wall_geometry=foundation.enum.ConductionWallGeometry.Planar  area=battery_cellH*battery_cellW m^2  thickness=endPlateThickness m  d_in=0.05 m  d_out=0.1 m  L=1 m  th_cond_min=10 W/(K*m)  th_cond=0.024 W/(m*K)  th_cond_TLU=[413, 401, 392, 383, 371, 357, 342] W/(K*m)  temp_TLU=[200, 273, 400, 600, 800, 1000, 1200] K  T_specify=off  T_priority=None  T=0 K  T_nominal_specify=off  T_nominal_value=1  T_nominal_unit=K  Q_specify=off  Q_priority=None  Q=0 W  Q_nominal_specify=off  Q_nominal_value=1  Q_nominal_unit=W
  plasticPlate : fl_lib/Thermal/Thermal Elements/Thermal Mass  mass_type=foundation.enum.constant_variable.constant  mass=battery_cellH*battery_cellW*endPlateThickness*44 kg  sp_heat=400 J/kg/K  mass_min=1e-6 kg  num_ports=foundation.enum.numPorts2.one  m_specify=off  m_priority=High  m=1 kg  m_nominal_specify=off  m_nominal_value=1  m_nominal_unit=kg  T_specify=off  T_priority=High  T=300 K  T_nominal_specify=off  T_nominal_value=1  T_nominal_unit=K  Q_specify=off  Q_priority=None  Q=0 W  Q_nominal_specify=off  Q_nominal_value=1  Q_nominal_unit=W
  amb : PMIOPort  Side=Left
  M3 : PMIOPort  Port=2  Side=Right
  connections:
  Conductive Heat Transfer1/LConn1 -- plasticPlate/LConn1 -- Conductive Heat Transfer/RConn1
  Conductive Heat Transfer/LConn1 -- M3/RConn1
  Conductive Heat Transfer1/RConn1 -- amb/RConn1

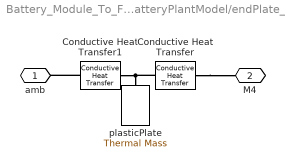
== system Battery_Module_To_FullPack_Grouped/BatteryPlantModel/endPlate_M4 ==
  Conductive Heat Transfer : fl_lib/Thermal/Thermal Elements/Conductive Heat Transfer  thermal_type=foundation.enum.ConstantVariableTabulated.Constant  wall_geometry=foundation.enum.ConductionWallGeometry.Planar  area=battery_cellH*battery_cellW m^2  thickness=endPlateThickness m  d_in=0.05 m  d_out=0.1 m  L=1 m  th_cond_min=10 W/(K*m)  th_cond=0.024 W/(m*K)  th_cond_TLU=[413, 401, 392, 383, 371, 357, 342] W/(K*m)  temp_TLU=[200, 273, 400, 600, 800, 1000, 1200] K  T_specify=off  T_priority=None  T=0 K  T_nominal_specify=off  T_nominal_value=1  T_nominal_unit=K  Q_specify=off  Q_priority=None  Q=0 W  Q_nominal_specify=off  Q_nominal_value=1  Q_nominal_unit=W
  Conductive Heat Transfer1 : fl_lib/Thermal/Thermal Elements/Conductive Heat Transfer  thermal_type=foundation.enum.ConstantVariableTabulated.Constant  wall_geometry=foundation.enum.ConductionWallGeometry.Planar  area=battery_cellH*battery_cellW m^2  thickness=endPlateThickness m  d_in=0.05 m  d_out=0.1 m  L=1 m  th_cond_min=10 W/(K*m)  th_cond=0.024 W/(m*K)  th_cond_TLU=[413, 401, 392, 383, 371, 357, 342] W/(K*m)  temp_TLU=[200, 273, 400, 600, 800, 1000, 1200] K  T_specify=off  T_priority=None  T=0 K  T_nominal_specify=off  T_nominal_value=1  T_nominal_unit=K  Q_specify=off  Q_priority=None  Q=0 W  Q_nominal_specify=off  Q_nominal_value=1  Q_nominal_unit=W
  plasticPlate : fl_lib/Thermal/Thermal Elements/Thermal Mass  mass_type=foundation.enum.constant_variable.constant  mass=battery_cellH*battery_cellW*endPlateThickness*44 kg  sp_heat=400 J/kg/K  mass_min=1e-6 kg  num_ports=foundation.enum.numPorts2.one  m_specify=off  m_priority=High  m=1 kg  m_nominal_specify=off  m_nominal_value=1  m_nominal_unit=kg  T_specify=off  T_priority=High  T=300 K  T_nominal_specify=off  T_nominal_value=1  T_nominal_unit=K  Q_specify=off  Q_priority=None  Q=0 W  Q_nominal_specify=off  Q_nominal_value=1  Q_nominal_unit=W
  amb : PMIOPort  Side=Left
  M4 : PMIOPort  Port=2  Side=Right
  connections:
  Conductive Heat Transfer1/LConn1 -- plasticPlate/LConn1 -- Conductive Heat Transfer/RConn1
  Conductive Heat Transfer/LConn1 -- M4/RConn1
  Conductive Heat Transfer1/RConn1 -- amb/RConn1
